simulink model "INS2_model"  (R2017a)
settings: Solver=ode4  StartTime=0.0  StopTime=30  FixedStep=0.01  RelTol=1e-3
values from neighbouring files (symbols this model uses):
  del_a_s = 10^-2 * del_K * n  -  M * n  +  del_a    [INS2_init.m]
  del_w_s = 10^-2 * del_K * w  -  M * w  +  eps    [INS2_init.m]
  n = [0 9.81 0]'    [INS2_init.m]
  sig_arw = ARW / sqrt(Ts)    [INS2_init.m]
  sig_larw = LARW / sqrt(Ts)    [INS2_init.m]
  sig_rrw = RRW / sqrt(Ts)    [INS2_init.m]
  sig_vrw = VRW / sqrt(Ts)    [INS2_init.m]
  Ts = 0.01    [INS2_init.m]
  w = [0 0 0]'    [INS2_init.m]
undefined symbols (not defined in the file or in its folder): datetime, posixtime
libraries: simulink x12, dspsrcs4 x6
settings Model: Creator=Alex  LastModifiedBy=Alex

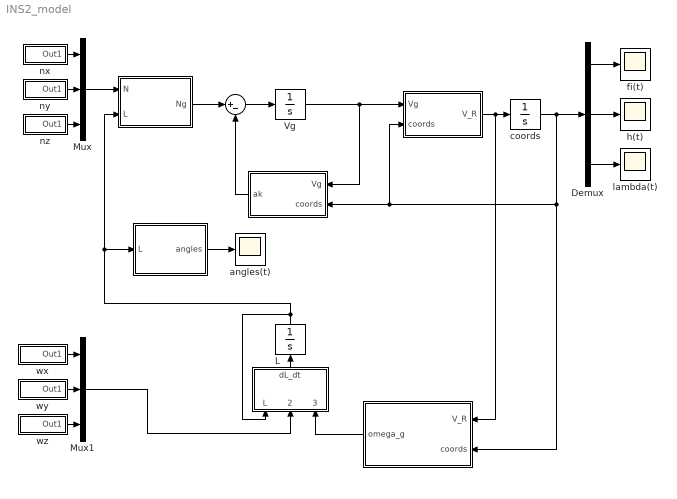
== system INS2_model ==
  " " : Sum  Inputs=|+-
  "  " : MATLAB Function  TreatAsAtomicUnit=on
  "   " : MATLAB Function  TreatAsAtomicUnit=on
  "    " : MATLAB Function  TreatAsAtomicUnit=on
  "     " : MATLAB Function  TreatAsAtomicUnit=on
  "      " : MATLAB Function  TreatAsAtomicUnit=on
  "       " : MATLAB Function  TreatAsAtomicUnit=on
  Demux : Demux  Outputs=3
  L : Integrator  InitialCondition=[1 0 0 0]
  Mux : Mux  Inputs=3
  Mux1 : Mux  Inputs=3
  Vg : Integrator  InitialCondition=[0 0 0]
  angles(t) : Scope
  coords : Integrator  InitialCondition=[0 0 0]
  fi(t) : Scope
  h(t) : Scope
  lambda(t) : Scope
  nx : Subsystem
  ny : Subsystem
  nz : Subsystem
  wx : Subsystem
  wy : Subsystem
  wz : Subsystem
  wires:
  Mux/1 -> "     "/1(N)
  " "/1 -> Vg/1
  "    "/1(ak) -> " "/2
  "      "/1(V_R) -> "  "/1(V_R), coords/1
  coords/1 -> "      "/2(coords), "    "/2(coords), "  "/2(coords), Demux/1
  wx/1(Out1) -> Mux1/1
  wy/1(Out1) -> Mux1/2
  wz/1(Out1) -> Mux1/3
  "  "/1(omega_g) -> "   "/3(omega_g)
  Mux1/1 -> "   "/2(omega)
  "       "/1(angles) -> angles(t)/1
  "   "/1(dL_dt) -> L/1
  L/1 -> "   "/1(L), "       "/1(L), "     "/2(L)
  Demux/1 -> fi(t)/1
  Demux/2 -> h(t)/1
  Demux/3 -> lambda(t)/1
  Vg/1 -> "    "/1(Vg), "      "/1(Vg)
  "     "/1(Ng) -> " "/1
  nx/1(Out1) -> Mux/1
  ny/1(Out1) -> Mux/2
  nz/1(Out1) -> Mux/3

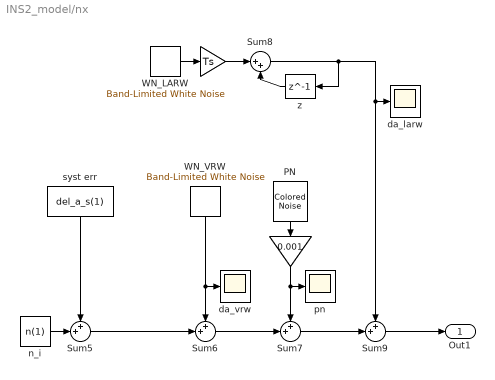
== system INS2_model/nx ==
  " " : Gain  Gain=0.001
  "  " : Gain  Gain=Ts
  " WN_LARW" : simulink/Sources/Band-Limited White Noise  Cov=sig_larw^2 * Ts  Ts=Ts  seed=[floor( posixtime( datetime ) ) + 2]
  " WN_VRW" : simulink/Sources/Band-Limited White Noise  Cov=sig_vrw^2 * Ts  Ts=Ts  seed=[floor( posixtime( datetime ) ) + 3]
  "PN " : dspsrcs4/Colored Noise  Color=pink  InverseFrequencyPower=1  NumChannels=1  OutputDataType=double  SamplesPerFrame=1  SampleTime=Ts  RandomStream=mt19937ar with seed  Seed=floor( posixtime( datetime ) ) + 1  SimulateUsing=Interpreted execution
      settings: SourceProductName=DSP System Toolbox  SourceProductBaseCode=DS
  Sum{5..7,9} (4 alike) : Sum  Inputs=++|
  Sum8 : Sum  Inputs=|++
  da_larw : Scope
  da_vrw : Scope
  n_i : Constant  Value=n(1)
  "pn " : Scope
  "syst err " : Constant  Value=del_a_s(1)
  "z " : Delay  DelayLength=1  InitialCondition=0
  Out1 : Outport
  wires:
  "PN "/1 -> " "/1
  " "/1 -> "pn "/1, Sum7/1
  Sum8/1 -> "z "/1, da_larw/1, Sum9/1
  "z "/1 -> Sum8/2
  Sum9/1 -> Out1/1
  Sum7/1 -> Sum9/2
  "syst err "/1 -> Sum5/1
  n_i/1 -> Sum5/2
  " WN_LARW"/1 -> "  "/1
  Sum5/1 -> Sum6/2
  " WN_VRW"/1 -> da_vrw/1, Sum6/1
  Sum6/1 -> Sum7/2
  "  "/1 -> Sum8/1

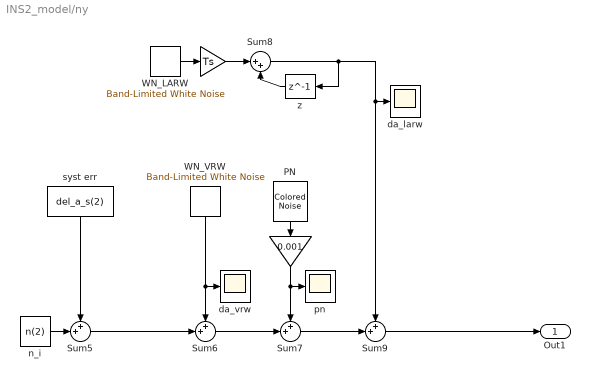
== system INS2_model/ny ==
  " " : Gain  Gain=0.001
  "  " : Gain  Gain=Ts
  " WN_LARW" : simulink/Sources/Band-Limited White Noise  Cov=sig_larw^2 * Ts  Ts=Ts  seed=[floor( posixtime( datetime ) ) + 2]
  " WN_VRW" : simulink/Sources/Band-Limited White Noise  Cov=sig_vrw^2 * Ts  Ts=Ts  seed=[floor( posixtime( datetime ) ) + 3]
  "PN " : dspsrcs4/Colored Noise  Color=pink  InverseFrequencyPower=1  NumChannels=1  OutputDataType=double  SamplesPerFrame=1  SampleTime=Ts  RandomStream=mt19937ar with seed  Seed=floor( posixtime( datetime ) ) + 1  SimulateUsing=Interpreted execution
      settings: SourceProductName=DSP System Toolbox  SourceProductBaseCode=DS
  Sum{5..7,9} (4 alike) : Sum  Inputs=++|
  Sum8 : Sum  Inputs=|++
  da_larw : Scope
  da_vrw : Scope
  n_i : Constant  Value=n(2)
  "pn " : Scope
  "syst err " : Constant  Value=del_a_s(2)
  "z " : Delay  DelayLength=1  InitialCondition=0
  Out1 : Outport
  wires:
  "  "/1 -> Sum8/1
  Sum6/1 -> Sum7/2
  " WN_VRW"/1 -> Sum6/1, da_vrw/1
  Sum5/1 -> Sum6/2
  " WN_LARW"/1 -> "  "/1
  n_i/1 -> Sum5/2
  "syst err "/1 -> Sum5/1
  Sum7/1 -> Sum9/2
  Sum9/1 -> Out1/1
  "z "/1 -> Sum8/2
  Sum8/1 -> Sum9/1, da_larw/1, "z "/1
  " "/1 -> Sum7/1, "pn "/1
  "PN "/1 -> " "/1

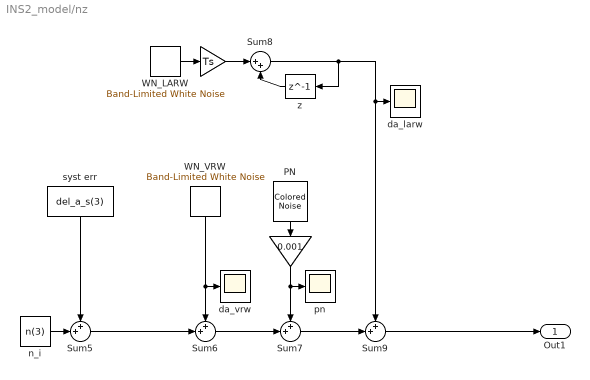
== system INS2_model/nz ==
  " " : Gain  Gain=0.001
  "  " : Gain  Gain=Ts
  " WN_LARW" : simulink/Sources/Band-Limited White Noise  Cov=sig_larw^2 * Ts  Ts=Ts  seed=[floor( posixtime( datetime ) ) + 2]
  " WN_VRW" : simulink/Sources/Band-Limited White Noise  Cov=sig_vrw^2 * Ts  Ts=Ts  seed=[floor( posixtime( datetime ) ) + 3]
  "PN " : dspsrcs4/Colored Noise  Color=pink  InverseFrequencyPower=1  NumChannels=1  OutputDataType=double  SamplesPerFrame=1  SampleTime=Ts  RandomStream=mt19937ar with seed  Seed=floor( posixtime( datetime ) ) + 1  SimulateUsing=Interpreted execution
      settings: SourceProductName=DSP System Toolbox  SourceProductBaseCode=DS
  Sum{5..7,9} (4 alike) : Sum  Inputs=++|
  Sum8 : Sum  Inputs=|++
  da_larw : Scope
  da_vrw : Scope
  n_i : Constant  Value=n(3)
  "pn " : Scope
  "syst err " : Constant  Value=del_a_s(3)
  "z " : Delay  DelayLength=1  InitialCondition=0
  Out1 : Outport
  wires:
  "PN "/1 -> " "/1
  " "/1 -> "pn "/1, Sum7/1
  Sum8/1 -> "z "/1, da_larw/1, Sum9/1
  "z "/1 -> Sum8/2
  Sum9/1 -> Out1/1
  Sum7/1 -> Sum9/2
  "syst err "/1 -> Sum5/1
  n_i/1 -> Sum5/2
  " WN_LARW"/1 -> "  "/1
  Sum5/1 -> Sum6/2
  " WN_VRW"/1 -> da_vrw/1, Sum6/1
  Sum6/1 -> Sum7/2
  "  "/1 -> Sum8/1

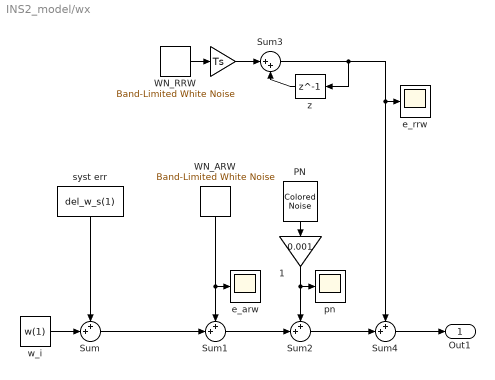
== system INS2_model/wx ==
  " 1" : Gain  Gain=0.001
  "      " : Gain  Gain=Ts
  " WN_ARW" : simulink/Sources/Band-Limited White Noise  Cov=sig_arw^2 * Ts  Ts=Ts  seed=[floor( posixtime( datetime ) )+1]
  " WN_RRW" : simulink/Sources/Band-Limited White Noise  Cov=sig_rrw^2 * Ts  Ts=Ts  seed=[floor( posixtime( datetime ) )]
  PN : dspsrcs4/Colored Noise  Color=pink  InverseFrequencyPower=1  NumChannels=1  OutputDataType=double  SamplesPerFrame=1  SampleTime=Ts  RandomStream=mt19937ar with seed  Seed=floor( posixtime( datetime ) )  SimulateUsing=Interpreted execution
      settings: SourceProductName=DSP System Toolbox  SourceProductBaseCode=DS
  Sum{,1..2,4} (4 alike) : Sum  Inputs=++|
  Sum3 : Sum  Inputs=|++
  e_arw : Scope
  e_rrw : Scope
  pn : Scope
  syst err : Constant  Value=del_w_s(1)
  w_i : Constant  Value=w(1)
  z : Delay  DelayLength=1  InitialCondition=0
  Out1 : Outport
  wires:
  Sum/1 -> Sum1/2
  syst err/1 -> Sum/1
  z/1 -> Sum3/2
  w_i/1 -> Sum/2
  Sum4/1 -> Out1/1
  Sum3/1 -> z/1, e_rrw/1, Sum4/1
  Sum2/1 -> Sum4/2
  "      "/1 -> Sum3/1
  Sum1/1 -> Sum2/2
  PN/1 -> " 1"/1
  " WN_RRW"/1 -> "      "/1
  " WN_ARW"/1 -> e_arw/1, Sum1/1
  " 1"/1 -> pn/1, Sum2/1

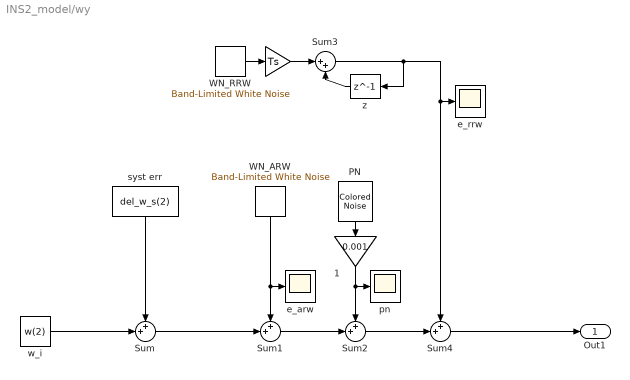
== system INS2_model/wy ==
  " 1" : Gain  Gain=0.001
  "      " : Gain  Gain=Ts
  " WN_ARW" : simulink/Sources/Band-Limited White Noise  Cov=sig_arw^2 * Ts  Ts=Ts  seed=[floor( posixtime( datetime ) )+1]
  " WN_RRW" : simulink/Sources/Band-Limited White Noise  Cov=sig_rrw^2 * Ts  Ts=Ts  seed=[floor( posixtime( datetime ) )]
  PN : dspsrcs4/Colored Noise  Color=pink  InverseFrequencyPower=1  NumChannels=1  OutputDataType=double  SamplesPerFrame=1  SampleTime=Ts  RandomStream=mt19937ar with seed  Seed=floor( posixtime( datetime ) )  SimulateUsing=Interpreted execution
      settings: SourceProductName=DSP System Toolbox  SourceProductBaseCode=DS
  Sum{,1..2,4} (4 alike) : Sum  Inputs=++|
  Sum3 : Sum  Inputs=|++
  e_arw : Scope
  e_rrw : Scope
  pn : Scope
  syst err : Constant  Value=del_w_s(2)
  w_i : Constant  Value=w(2)
  z : Delay  DelayLength=1  InitialCondition=0
  Out1 : Outport
  wires:
  " 1"/1 -> Sum2/1, pn/1
  " WN_ARW"/1 -> Sum1/1, e_arw/1
  " WN_RRW"/1 -> "      "/1
  PN/1 -> " 1"/1
  Sum1/1 -> Sum2/2
  "      "/1 -> Sum3/1
  Sum2/1 -> Sum4/2
  Sum3/1 -> Sum4/1, e_rrw/1, z/1
  Sum4/1 -> Out1/1
  w_i/1 -> Sum/2
  z/1 -> Sum3/2
  syst err/1 -> Sum/1
  Sum/1 -> Sum1/2

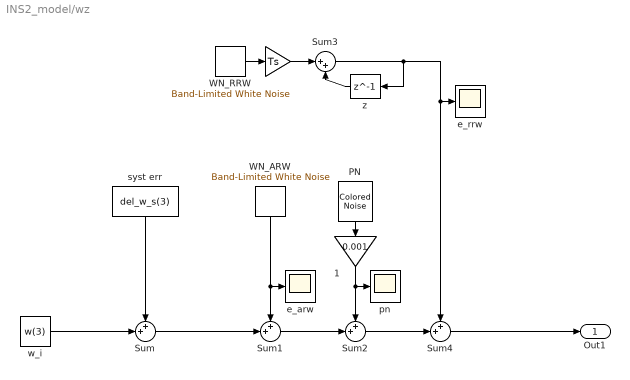
== system INS2_model/wz ==
  " 1" : Gain  Gain=0.001
  "      " : Gain  Gain=Ts
  " WN_ARW" : simulink/Sources/Band-Limited White Noise  Cov=sig_arw^2 * Ts  Ts=Ts  seed=[floor( posixtime( datetime ) )+1]
  " WN_RRW" : simulink/Sources/Band-Limited White Noise  Cov=sig_rrw^2 * Ts  Ts=Ts  seed=[floor( posixtime( datetime ) )]
  PN : dspsrcs4/Colored Noise  Color=pink  InverseFrequencyPower=1  NumChannels=1  OutputDataType=double  SamplesPerFrame=1  SampleTime=Ts  RandomStream=mt19937ar with seed  Seed=floor( posixtime( datetime ) )  SimulateUsing=Interpreted execution
      settings: SourceProductName=DSP System Toolbox  SourceProductBaseCode=DS
  Sum{,1..2,4} (4 alike) : Sum  Inputs=++|
  Sum3 : Sum  Inputs=|++
  e_arw : Scope
  e_rrw : Scope
  pn : Scope
  syst err : Constant  Value=del_w_s(3)
  w_i : Constant  Value=w(3)
  z : Delay  DelayLength=1  InitialCondition=0
  Out1 : Outport
  wires:
  Sum/1 -> Sum1/2
  syst err/1 -> Sum/1
  z/1 -> Sum3/2
  w_i/1 -> Sum/2
  Sum4/1 -> Out1/1
  Sum3/1 -> z/1, e_rrw/1, Sum4/1
  Sum2/1 -> Sum4/2
  "      "/1 -> Sum3/1
  Sum1/1 -> Sum2/2
  PN/1 -> " 1"/1
  " WN_RRW"/1 -> "      "/1
  " WN_ARW"/1 -> e_arw/1, Sum1/1
  " 1"/1 -> pn/1, Sum2/1

== matlab function INS2_model/     ==
  data: Vg input size=3; ak output size=3; coords input size=3
function ak  = fcn(Vg,coords)

    R = 6371100;
    U = 0.00007292115078;
    g = 9.81;
    
    ak = [
          (Vg(3)^2*tan(coords(1))/R) + (Vg(1)*Vg(2)/R) + (2*U*Vg(3)*sin(coords(1)));
          (-Vg(3)^2/R)-(Vg(1)^2/R) - (2*U*Vg(3)*cos(coords(1))) + g;
          (Vg(3)*Vg(2)/R) - (Vg(3)*Vg(1)*tan(coords(1))/R) + 2*(U*Vg(2)*cos(coords(1)) - U*Vg(1)*sin(coords(1)))
          ];
end

== matlab function INS2_model/      ==
  data: N input size=3; Ng output size=3; L input size=4
function Ng = fcn(N, L)

    N = [ 0; N ];
    
    L_conj = [ L(1); -L(2); -L(3); -L(4) ];

    Ng_0 = toMatrix( toMatrix(L) * N ) * L_conj
    
    Ng = Ng_0(2:end) % remove 0
end

== matlab function INS2_model/    ==
  data: L input size=4; dL_dt output size=4; omega input size=3; omega_g input size=3
function dL_dt = fcn( L, omega, omega_g)
    
    sigma   = [ 0; omega ];  
    sigma_g = [ 0; omega_g ];

    dL_dt = (toMatrix(L) * sigma  -  toMatrix(sigma_g) * L  +  L * (1 - sum(L.^2))) ./ 2;
end

== matlab function INS2_model/       ==
  data: Vg input size=3; V_R output size=3; coords input size=3
function V_R  = fcn(Vg,coords)

    R = 6371100;
    
    V_R = [
            Vg(1)/R;
            Vg(2);
            Vg(3)/(R*cos(coords(1)))
            ];
end

== matlab function INS2_model/   ==
  data: V_R input size=3; omega_g output size=3; coords input size=3
function omega_g  = fcn(V_R,coords)

    U = 0.00007292115078;
    
    omega_g = [
              (U+V_R(3))*cos(coords(1));
              (U+V_R(3))*sin(coords(1));
              -V_R(1)
              ];
end

== matlab function INS2_model/        ==
  data: angles output size=3; L input size=4
function angles = fcn(L)

    psi   = atan( -(2*L(2)*L(4)-2*L(1)*L(3))/(2*L(2)^2+2*L(1)^2-1) );
    theta = asin(2*L(2)*L(3)+2*L(1)*L(4));
    gamma = atan( -(2*L(3)*L(4)-2*L(1)*L(2))/(2*L(1)^2+2*L(3)^2-1) );

    angles = [psi; theta; gamma];
end
